simulink model "gm_soc_dvbs2_fpga"  (R2025b)
settings: Solver=VariableStepAuto  StartTime=0.0  StopTime=10.0  RelTol=1e-3
InitFcn:
  | soc_dvbs2_init;
undefined symbols (not defined in the file or in its folder): Add, coefficientsLog, coefficientsSqrt1, coefficientsSqrt2, dataBits, Deinterleaver, designMultirateFIR, noisePow, Shift, Short, soc_dvbs2_designFIRFilter, soc_dvbs2_txPacketBits, syncWord, txDataOut, txFiltCoeff, XData
libraries: simulink x304, hdlsllib x265, dspsigops x15, dsphdlfiltering2 x8, hdlmdlgenlib x6, dsphdlsigops2 x5, commseqgen3 x5, dsphdlmathfun2 x3, hwlogicconnlib x2, whdledac x2, commhdlcrc x2, whdlutilities x1
(part 24 of 36)

== system gm_soc_dvbs2_fpga/DVBS2/DVBS2 TxRx/Channel/AWGN Generator/Unit Variance Gaussian Noise/SinCos/Sine HDL Optimized1/Look-Up Table ==
  In1 : Inport
  Look-Up Table : Lookup_n-D  NumberOfTableDimensions=1  LookupTableObject=''  BreakpointsSpecification=Even spacing  BreakpointsForDimension1=XData  BreakpointsForDimension1FirstPoint="fi(0,0,12,0,\"hex\",\"000\")"  BreakpointsForDimension1Spacing="fi(0,0,12,0,\"hex\",\"001\")"  IndexSearchMethod=Evenly spaced points  Table="fi(\"numerictype\",numerictype(0,15,15),\"Value\",\"[0 0.00152587890625 0.003082275390625 0.004608154296875 0.006134033203125 0.007659912109375 0.00921630859375 0.0107421875 0.01226806640625 0.0137939453125 0.015350341796875 0.016876220703125 0.018402099609375 0.019927978515625 0.021484375 0.02301025390625 0.0245361328125 0.02606201171875 0.027618408203125 0.029144287109375 0.030670166015625 0.032196044921875 0.03375244140625 0.0352783203125 0.03680419921875 0.038330078125 0.039886474609375 0.041412353515625 0.042938232421875 0.044464111328125 0.045989990234375 0.04754638671875 0.049072265625 0.05059814453125 0.0521240234375 0.05364990234375 0.055206298828125 0.056732177734375 0.058258056640625 0.059783935546875 0.061309814453125 0.0628662109375 0.06439208984375 0.06591796875 0.06744384765625 0.0689697265625 0.07049560546875 0.072021484375 0.073577880859375 0.075103759765625 0.076629638671875 0.078155517578125 0.079681396484375 0.081207275390625 0.082733154296875 0.084259033203125 0.085784912109375 0.087310791015625 0.0888671875 0.09039306640625 0.0919189453125 0.09344482421875 0.094970703125 0.09649658203125 0.0980224609375 0.09954833984375 0.10107421875 0.10260009765625 0.1041259765625 0.10565185546875 0.107177734375 0.10870361328125 0.1102294921875 0.11175537109375 0.11328125 0.11480712890625 0.1163330078125 0.117828369140625 0.119354248046875 0.120880126953125 0.122406005859375 0.123931884765625 0.125457763671875 0.126983642578125 0.128509521484375 0.1300048828125 0.13153076171875 0.133056640625 0.13458251953125 0.1361083984375 0.13763427734375 0.139129638671875 0.140655517578125 0.142181396484375 0.143707275390625 0.14520263671875 0.146728515625 0.14825439453125 0.149749755859375 0.151275634765625 0.152801513671875 0.154327392578125 0.15582275390625 0.1573486328125 0.158843994140625 0.160369873046875 0.161895751953125 0.16339111328125 0.1649169921875 0.166412353515625 0.167938232421875 0.169464111328125 0.17095947265625 0.1724853515625 0.173980712890625 0.175506591796875 0.177001953125 0.17852783203125 0.180023193359375 0.1815185546875 0.18304443359375 0.184539794921875 0.186065673828125 0.18756103515625 0.189056396484375 0.190582275390625 0.19207763671875 0.193572998046875 0.195098876953125 0.19659423828125 0.198089599609375 0.199615478515625 0.20111083984375 0.202606201171875 0.2041015625 0.205596923828125 0.207122802734375 0.2086181640625 0.210113525390625 0.21160888671875 0.213104248046875 0.214599609375 0.216094970703125 0.21759033203125 0.2191162109375 0.220611572265625 0.22210693359375 0.223602294921875 0.22509765625 0.226593017578125 0.228057861328125 0.22955322265625 0.231048583984375 0.2325439453125 0.234039306640625 0.23553466796875 0.237030029296875 0.238525390625 0.239990234375 0.241485595703125 0.24298095703125 0.244476318359375 0.245941162109375 0.2474365234375 0.248931884765625 0.25042724609375 0.25189208984375 0.253387451171875 0.254852294921875 0.25634765625 0.257843017578125 0.259307861328125 0.26080322265625 0.26226806640625 0.263763427734375 0.265228271484375 0.2667236328125 0.2681884765625 0.2696533203125 0.271148681640625 0.272613525390625 0.27410888671875 0.27557373046875 0.27703857421875 0.278533935546875 0.279998779296875 0.281463623046875 0.282928466796875 0.284393310546875 0.285888671875 0.287353515625 0.288818359375 0.290283203125 0.291748046875 0.293212890625 0.294677734375 0.296142578125 0.297607421875 0.299072265625 0.300537109375 0.302001953125 0.303466796875 0.304931640625 0.306396484375 0.307861328125 0.309295654296875 0.310760498046875 0.312225341796875 0.313690185546875 0.31512451171875 0.31658935546875 0.31805419921875 0.319488525390625 0.320953369140625 0.322418212890625 0.3238525390625 0.3253173828125 0.326751708984375 0.328216552734375 0.32965087890625 0.33111572265625 0.332550048828125 0.334014892578125 0.33544921875 0.336883544921875 0.338348388671875 0.33978271484375 0.341217041015625 0.3426513671875 0.3441162109375 0.345550537109375 0.34698486328125 0.348419189453125 0.349853515625 0.351287841796875 0.35272216796875 ...(+13376 chars)]\")"  TableDataTypeStr=fixdt(0,15,15)  InterpMethod=Flat  ExtrapMethod=Clip  OutDataTypeStr=fixdt(1,16,15)
  Look-Up Table_pd1 : Delay  DelayLength=1
  Out1 : Outport
  wires:
  In1/1 -> Look-Up Table/1
  Look-Up Table_pd1/1 -> Out1/1
  Look-Up Table/1 -> Look-Up Table_pd1/1

== system gm_soc_dvbs2_fpga/DVBS2/DVBS2 TxRx/Channel/AWGN Generator/Unit Variance Gaussian Noise/SinCos/Sine HDL Optimized2/Look-Up Table ==
  In1 : Inport
  Look-Up Table : Lookup_n-D  NumberOfTableDimensions=1  LookupTableObject=''  BreakpointsSpecification=Even spacing  BreakpointsForDimension1=XData  BreakpointsForDimension1FirstPoint="fi(0,0,12,0,\"hex\",\"000\")"  BreakpointsForDimension1Spacing="fi(0,0,12,0,\"hex\",\"001\")"  IndexSearchMethod=Evenly spaced points  Table="fi(\"numerictype\",numerictype(0,15,15),\"Value\",\"[0 0.00152587890625 0.003082275390625 0.004608154296875 0.006134033203125 0.007659912109375 0.00921630859375 0.0107421875 0.01226806640625 0.0137939453125 0.015350341796875 0.016876220703125 0.018402099609375 0.019927978515625 0.021484375 0.02301025390625 0.0245361328125 0.02606201171875 0.027618408203125 0.029144287109375 0.030670166015625 0.032196044921875 0.03375244140625 0.0352783203125 0.03680419921875 0.038330078125 0.039886474609375 0.041412353515625 0.042938232421875 0.044464111328125 0.045989990234375 0.04754638671875 0.049072265625 0.05059814453125 0.0521240234375 0.05364990234375 0.055206298828125 0.056732177734375 0.058258056640625 0.059783935546875 0.061309814453125 0.0628662109375 0.06439208984375 0.06591796875 0.06744384765625 0.0689697265625 0.07049560546875 0.072021484375 0.073577880859375 0.075103759765625 0.076629638671875 0.078155517578125 0.079681396484375 0.081207275390625 0.082733154296875 0.084259033203125 0.085784912109375 0.087310791015625 0.0888671875 0.09039306640625 0.0919189453125 0.09344482421875 0.094970703125 0.09649658203125 0.0980224609375 0.09954833984375 0.10107421875 0.10260009765625 0.1041259765625 0.10565185546875 0.107177734375 0.10870361328125 0.1102294921875 0.11175537109375 0.11328125 0.11480712890625 0.1163330078125 0.117828369140625 0.119354248046875 0.120880126953125 0.122406005859375 0.123931884765625 0.125457763671875 0.126983642578125 0.128509521484375 0.1300048828125 0.13153076171875 0.133056640625 0.13458251953125 0.1361083984375 0.13763427734375 0.139129638671875 0.140655517578125 0.142181396484375 0.143707275390625 0.14520263671875 0.146728515625 0.14825439453125 0.149749755859375 0.151275634765625 0.152801513671875 0.154327392578125 0.15582275390625 0.1573486328125 0.158843994140625 0.160369873046875 0.161895751953125 0.16339111328125 0.1649169921875 0.166412353515625 0.167938232421875 0.169464111328125 0.17095947265625 0.1724853515625 0.173980712890625 0.175506591796875 0.177001953125 0.17852783203125 0.180023193359375 0.1815185546875 0.18304443359375 0.184539794921875 0.186065673828125 0.18756103515625 0.189056396484375 0.190582275390625 0.19207763671875 0.193572998046875 0.195098876953125 0.19659423828125 0.198089599609375 0.199615478515625 0.20111083984375 0.202606201171875 0.2041015625 0.205596923828125 0.207122802734375 0.2086181640625 0.210113525390625 0.21160888671875 0.213104248046875 0.214599609375 0.216094970703125 0.21759033203125 0.2191162109375 0.220611572265625 0.22210693359375 0.223602294921875 0.22509765625 0.226593017578125 0.228057861328125 0.22955322265625 0.231048583984375 0.2325439453125 0.234039306640625 0.23553466796875 0.237030029296875 0.238525390625 0.239990234375 0.241485595703125 0.24298095703125 0.244476318359375 0.245941162109375 0.2474365234375 0.248931884765625 0.25042724609375 0.25189208984375 0.253387451171875 0.254852294921875 0.25634765625 0.257843017578125 0.259307861328125 0.26080322265625 0.26226806640625 0.263763427734375 0.265228271484375 0.2667236328125 0.2681884765625 0.2696533203125 0.271148681640625 0.272613525390625 0.27410888671875 0.27557373046875 0.27703857421875 0.278533935546875 0.279998779296875 0.281463623046875 0.282928466796875 0.284393310546875 0.285888671875 0.287353515625 0.288818359375 0.290283203125 0.291748046875 0.293212890625 0.294677734375 0.296142578125 0.297607421875 0.299072265625 0.300537109375 0.302001953125 0.303466796875 0.304931640625 0.306396484375 0.307861328125 0.309295654296875 0.310760498046875 0.312225341796875 0.313690185546875 0.31512451171875 0.31658935546875 0.31805419921875 0.319488525390625 0.320953369140625 0.322418212890625 0.3238525390625 0.3253173828125 0.326751708984375 0.328216552734375 0.32965087890625 0.33111572265625 0.332550048828125 0.334014892578125 0.33544921875 0.336883544921875 0.338348388671875 0.33978271484375 0.341217041015625 0.3426513671875 0.3441162109375 0.345550537109375 0.34698486328125 0.348419189453125 0.349853515625 0.351287841796875 0.35272216796875 ...(+13376 chars)]\")"  TableDataTypeStr=fixdt(0,15,15)  InterpMethod=Flat  ExtrapMethod=Clip  OutDataTypeStr=fixdt(1,16,15)
  Look-Up Table_pd1 : Delay  DelayLength=1
  Out1 : Outport
  wires:
  In1/1 -> Look-Up Table/1
  Look-Up Table_pd1/1 -> Out1/1
  Look-Up Table/1 -> Look-Up Table_pd1/1

== system gm_soc_dvbs2_fpga/DVBS2/DVBS2 TxRx/Channel/AWGN Generator/Unit Variance Gaussian Noise/SqrtImplementation/SqrtEval/FunctionEvaluation ==
  x_f : Inport  OutDataTypeStr=fixdt(0, 31, 24)  PortDimensions=1  SampleTime=6.25e-08
  passIn : Inport  Port=2  OutDataTypeStr=fixdt(1, 9, 0)  PortDimensions=1  SampleTime=6.25e-08
  exp_fIn : Inport  Port=3  OutDataTypeStr=int8  PortDimensions=1  SampleTime=6.25e-08
  1-D Lookup Table : Subsystem
  1-D Lookup Table1 : Subsystem
  1-D Lookup Table2 : Subsystem
  1-D Lookup Table3 : Subsystem
  Add : Sum  OutDataTypeStr=fixdt(0, 17, 13)  AccumDataTypeStr=fixdt(1, 44, 36)  SampleTime=6.25e-08
  Add1 : Sum  OutDataTypeStr=fixdt(0, 17, 13)  AccumDataTypeStr=fixdt(0, 17, 13)  SampleTime=6.25e-08
  Constant : Constant  OutDataTypeStr=uint8  SampleTime=6.25e-08
  Constant1 : Constant  Value=2  OutDataTypeStr=uint8  SampleTime=6.25e-08
  Constant2 : Constant  Value=64  OutDataTypeStr=uint8  SampleTime=6.25e-08
  Data Type Conversion : DataTypeConversion  OutDataTypeStr=uint8  SampleTime=6.25e-08  SaturateOnIntegerOverflow=off  RndMeth=Floor
  Data Type Conversion1 : DataTypeConversion  OutDataTypeStr=uint8  SampleTime=6.25e-08  SaturateOnIntegerOverflow=off  RndMeth=Floor
  Delay{,1..7,9..10,13..14} (12 alike) : Delay  DelayLength=double(1)  InitialCondition=0  SampleTime=6.25e-08
  Delay{8,11..12,15..25} (14 alike) : Delay  DelayLength=double(2)  InitialCondition=0  SampleTime=6.25e-08
  Product : Product  Inputs=**  OutDataTypeStr=fixdt(1, 44, 36)  SampleTime=6.25e-08
  Product1 : Product  Inputs=**  OutDataTypeStr=fixdt(1, 44, 36)  SampleTime=6.25e-08
  Shift Arithmetic1 : ArithShift  BitShiftNumber=double(0)  BinPtShiftNumber=double(6)
  Shift Arithmetic2 : ArithShift  BitShiftNumber=double(0)  BinPtShiftNumber=double(5)
  Subtract : Sum  Inputs=+-  OutDataTypeStr=fixdt(1, 33, 24)  AccumDataTypeStr=fixdt(1, 33, 24)  SampleTime=6.25e-08
  Subtract1 : Sum  Inputs=+-  OutDataTypeStr=fixdt(0, 31, 24)  AccumDataTypeStr=fixdt(0, 31, 24)  SampleTime=6.25e-08
  Switch : Switch  Criteria=u2 ~= 0  Threshold="fi(0,1,9,0,\"hex\",\"000\")"  OutDataTypeStr=fixdt(0, 17, 13)  SampleTime=6.25e-08  SaturateOnIntegerOverflow=off  InputSameDT=off
  Switch1 : Switch  Criteria=u2 > Threshold  Threshold="fi(0,0,8,0,\"hex\",\"3f\")"  OutDataTypeStr=uint8  SampleTime=6.25e-08  SaturateOnIntegerOverflow=off  InputSameDT=off
  Switch2 : Switch  Criteria=u2 > Threshold  Threshold="fi(0,0,8,0,\"hex\",\"3f\")"  OutDataTypeStr=int8  SampleTime=6.25e-08  SaturateOnIntegerOverflow=off  InputSameDT=off
  y_f : Outport  SampleTime=6.25e-08
  passOut : Outport  Port=2  SampleTime=6.25e-08
  exp_fOut : Outport  Port=3  SampleTime=6.25e-08
  wires:
  Constant1/1 -> Subtract1/2
  Constant/1 -> Subtract/2
  Constant2/1 -> Switch2/1, Switch1/1
  exp_fIn/1 -> Delay7/1
  Shift Arithmetic2/1 -> Data Type Conversion1/1
  Subtract1/1 -> Shift Arithmetic2/1
  Subtract/1 -> Shift Arithmetic1/1
  x_f/1 -> Delay4/1, Subtract1/1, Delay/1, Subtract/1
  Delay7/1 -> Delay15/1
  Delay16/1 -> Add/1
  Delay/1 -> Delay8/1
  Delay15/1 -> Delay21/1
  Switch/1 -> y_f/1
  Shift Arithmetic1/1 -> Data Type Conversion/1
  Delay2/1 -> 1-D Lookup Table1/1(In1)
  Delay4/1 -> Delay12/1
  Delay21/1 -> Delay25/1
  Delay8/1 -> Product/1
  passIn/1 -> Delay3/1
  Data Type Conversion/1 -> Switch1/3, Switch1/2
  Switch1/1 -> Delay2/1, Delay1/1
  Data Type Conversion1/1 -> Switch2/3, Switch2/2
  Delay18/1 -> Delay23/1
  Delay25/1 -> exp_fOut/1
  Delay12/1 -> Product1/1
  Switch2/1 -> Delay6/1, Delay5/1
  Delay17/1 -> Add/2
  Delay1/1 -> 1-D Lookup Table/1(In1)
  Product/1 -> Delay16/1
  Delay5/1 -> 1-D Lookup Table2/1(In1)
  1-D Lookup Table/1(Out1) -> Delay9/1
  Delay6/1 -> 1-D Lookup Table3/1(In1)
  1-D Lookup Table2/1(Out1) -> Delay13/1
  1-D Lookup Table1/1(Out1) -> Delay10/1
  1-D Lookup Table3/1(Out1) -> Delay14/1
  Product1/1 -> Delay19/1
  Delay9/1 -> Product/2
  Delay10/1 -> Delay17/1
  Delay13/1 -> Product1/2
  Delay14/1 -> Delay20/1
  Delay19/1 -> Add1/1
  Delay3/1 -> Delay11/1
  Delay20/1 -> Add1/2
  Delay11/1 -> Delay18/1
  Add/1 -> Delay22/1
  Add1/1 -> Delay24/1
  Delay22/1 -> Switch/1
  Delay24/1 -> Switch/3
  Delay23/1 -> passOut/1, Switch/2

== system gm_soc_dvbs2_fpga/DVBS2/DVBS2 TxRx/Channel/AWGN Generator/Unit Variance Gaussian Noise/SqrtImplementation/SqrtEval/RangeReconstruction ==
  y_f : Inport  OutDataTypeStr=fixdt(0, 17, 13)  PortDimensions=1  SampleTime=6.25e-08
  pass : Inport  Port=2  OutDataTypeStr=fixdt(1, 9, 0)  PortDimensions=1  SampleTime=6.25e-08
  exp_f : Inport  Port=3  OutDataTypeStr=int8  PortDimensions=1  SampleTime=6.25e-08
  Add : Sum  OutDataTypeStr=int8  AccumDataTypeStr=int8
  Constant : Constant  OutDataTypeStr=int8  SampleTime=-1
  Delay{1..3,8} (4 alike) : Delay
  Delay{4..7,9..12} (8 alike) : Delay  DelayLength=1
  Gain : Gain  Gain=-1  OutDataTypeStr=int8
  Shift Arithmetic : ArithShift  BitShiftNumber=1
  Shift Arithmetic1 : ArithShift  BitShiftNumberSource=Input port  BitShiftNumber=8
      settings: InputPortMap=u0,p1
  Switch : Switch  Criteria=u2 ~= 0  OutDataTypeStr=int8  SaturateOnIntegerOverflow=off  InputSameDT=off
  f : Outport  SampleTime=6.25e-08
  wires:
  y_f/1 -> Delay9/1
  Delay12/1 -> Delay6/1
  Delay11/1 -> Delay7/1
  Delay2/1 -> Gain/1
  pass/1 -> Delay11/1
  Delay10/1 -> Add/2
  Constant/1 -> Add/1
  exp_f/1 -> Delay12/1, Delay10/1
  Delay4/1 -> Switch/1
  Delay6/1 -> Switch/3
  Add/1 -> Delay4/1
  Delay7/1 -> Switch/2
  Switch/1 -> Shift Arithmetic/1
  Delay9/1 -> Delay5/1
  Shift Arithmetic/1 -> Delay2/1
  Delay5/1 -> Delay3/1
  Delay3/1 -> Delay1/1
  Gain/1 -> Delay8/1
  Delay1/1 -> Shift Arithmetic1/1
  Shift Arithmetic1/1 -> f/1
  Delay8/1 -> Shift Arithmetic1/2

== system gm_soc_dvbs2_fpga/DVBS2/DVBS2 TxRx/Channel/AWGN Generator/Unit Variance Gaussian Noise/SqrtImplementation/SqrtEval/RangeReduction ==
  note: Range of x_f=[1,4)
  u : Inport  OutDataTypeStr=fixdt(0, 31, 24)  PortDimensions=1  SampleTime=6.25e-08
  Add : Sum  Inputs=+-  OutDataTypeStr=int8
  Constant : Constant  Value=5  OutDataTypeStr=uint8  SampleTime=-1
  Data Type Conversion : DataTypeConversion  OutDataTypeStr=fixdt(0,38,31)  SaturateOnIntegerOverflow=off  RndMeth=Floor
  Delay{1..20} (20 alike) : Delay  DelayLength=1
  Shift Arithmetic : ArithShift  BitShiftNumberSource=Input port  BitShiftNumber=8
      settings: InputPortMap=u0,p1
  Shift Arithmetic1 : ArithShift  BitShiftNumber=1  BitShiftDirection=Right
  Shift Arithmetic2 : ArithShift  BitShiftNumber=6  BitShiftDirection=Right
  Shift Arithmetic3 : ArithShift  BitShiftNumber=1  BitShiftDirection=Right
  Shift Arithmetic4 : ArithShift  BitShiftNumber=1  BitShiftDirection=Left
  Subtract : Sum  Inputs=+-  OutDataTypeStr=fixdt(1, 9, 0)
  Switch : Switch  Criteria=u2 ~= 0  OutDataTypeStr=fixdt(0, 31, 24)  SaturateOnIntegerOverflow=off  InputSameDT=off
  leadingZeroDetector : MATLAB Function  TreatAsAtomicUnit=on
  x_f : Outport  SampleTime=6.25e-08
  pass : Outport  Port=2  SampleTime=6.25e-08
  exp_f : Outport  Port=3  SampleTime=6.25e-08  VectorParamsAs1DForOutWhenUnconnected=off
  wires:
  u/1 -> Data Type Conversion/1, Delay3/1
  Delay20/1 -> leadingZeroDetector/1(x)
  Delay8/1 -> Subtract/1
  Delay19/1 -> Delay13/1
  Delay9/1 -> Subtract/2
  Delay2/1 -> Delay19/1
  Delay3/1 -> Delay2/1
  Shift Arithmetic2/1 -> Delay20/1
  Shift Arithmetic4/1 -> Delay9/1
  Data Type Conversion/1 -> Shift Arithmetic2/1
  leadingZeroDetector/1(exp_f) -> Delay4/1
  Delay16/1 -> Shift Arithmetic4/1
  Constant/1 -> Add/1
  Delay4/1 -> Add/2
  Delay13/1 -> Shift Arithmetic/1
  Shift Arithmetic3/1 -> Delay16/1
  Add/1 -> Delay18/1
  Delay10/1 -> Delay7/1
  Delay18/1 -> Shift Arithmetic3/1, Delay15/1, Delay14/1, Delay17/1
  Delay14/1 -> Shift Arithmetic/2
  Delay1/1 -> Switch/1
  Delay17/1 -> Delay10/1
  Delay15/1 -> Delay8/1
  Subtract/1 -> Delay6/1
  Shift Arithmetic/1 -> Delay11/1, Delay12/1
  Delay7/1 -> exp_f/1
  Delay12/1 -> Shift Arithmetic1/1
  Shift Arithmetic1/1 -> Delay1/1
  Delay11/1 -> Delay5/1
  Delay5/1 -> Switch/3
  Delay6/1 -> Switch/2, pass/1
  Switch/1 -> x_f/1

== system gm_soc_dvbs2_fpga/DVBS2/DVBS2 TxRx/Channel/AWGN Generator/Unit Variance Gaussian Noise/logImplementation/log/FunctionEvaluation ==
  x_e : Inport  OutDataTypeStr=fixdt(0, 49, 48)  PortDimensions=1  SampleTime=6.25e-08
  exp_eIn : Inport  Port=2  OutDataTypeStr=uint8  PortDimensions=1  SampleTime=6.25e-08
  1-D Lookup Table : Lookup_n-D  NumberOfTableDimensions=1  LookupTableObject=''  BreakpointsForDimension1=0:255  BreakpointsForDimension1FirstPoint=10  BreakpointsForDimension2FirstPoint=10  BreakpointsForDimension1Spacing=12  BreakpointsForDimension2Spacing=12  IndexSearchMethod=Evenly spaced points  Table=coefficientsLog(:,1)  InterpMethod=Flat  InternalRulePriority=Speed  OutDataTypeStr=fixdt(1,16,15)  RndMeth=Simplest
  1-D Lookup Table1 : Lookup_n-D  NumberOfTableDimensions=1  LookupTableObject=''  BreakpointsForDimension1=0:255  BreakpointsForDimension1FirstPoint=10  BreakpointsForDimension2FirstPoint=10  BreakpointsForDimension1Spacing=12  BreakpointsForDimension2Spacing=12  IndexSearchMethod=Evenly spaced points  Table=coefficientsLog(:,2)  InterpMethod=Flat  InternalRulePriority=Speed  OutDataTypeStr=fixdt(1,16,14)  RndMeth=Simplest
  1-D Lookup Table2 : Lookup_n-D  NumberOfTableDimensions=1  LookupTableObject=''  BreakpointsForDimension1=0:255  BreakpointsForDimension1FirstPoint=10  BreakpointsForDimension2FirstPoint=10  BreakpointsForDimension1Spacing=12  BreakpointsForDimension2Spacing=12  IndexSearchMethod=Evenly spaced points  Table=coefficientsLog(:,3)  InterpMethod=Flat  InternalRulePriority=Speed  OutDataTypeStr=fixdt(1,32,30)  RndMeth=Simplest
  Add : Sum  OutDataTypeStr=fixdt(1, 16, 14)  AccumDataTypeStr=fixdt(1, 18, 15)  SampleTime=6.25e-08
  Add1 : Sum  OutDataTypeStr=fixdt(1, 31, 27)  AccumDataTypeStr=fixdt(1, 35, 30)  SampleTime=6.25e-08
  Data Type Conversion : DataTypeConversion  OutDataTypeStr=uint8  SampleTime=6.25e-08  SaturateOnIntegerOverflow=off  RndMeth=Floor
  Data Type Conversion1 : DataTypeConversion  OutDataTypeStr=fixdt(0, 16, 15)  SampleTime=6.25e-08  SaturateOnIntegerOverflow=off  RndMeth=Floor
  Delay1 : Delay  DelayLength=double(1)  InitialCondition=0  SampleTime=6.25e-08
  Delay{3..30} (28 alike) : Delay  DelayLength=double(2)  InitialCondition=0  SampleTime=6.25e-08
  Delay2 : Delay  DelayLength=double(1)  InitialCondition=0  SampleTime=6.25e-08
  Product : Product  Inputs=**  OutDataTypeStr=fixdt(1, 32, 30)  SampleTime=6.25e-08
  Product1 : Product  Inputs=**  OutDataTypeStr=fixdt(1, 32, 29)  SampleTime=6.25e-08
  Product1_out_dtc : DataTypeConversion  OutDataTypeStr=fixdt(1, 31, 27)  SampleTime=6.25e-08  SaturateOnIntegerOverflow=off  RndMeth=Floor
  Product_out_dtc : DataTypeConversion  OutDataTypeStr=fixdt(1, 16, 15)  SampleTime=6.25e-08  SaturateOnIntegerOverflow=off  RndMeth=Floor
  Shift Arithmetic1 : ArithShift  BitShiftNumber=double(0)  BinPtShiftNumber=double(8)
  y_e : Outport  SampleTime=6.25e-08
  exp_eOut : Outport  Port=2  SampleTime=6.25e-08
  wires:
  Delay10/1 -> Add/1
  x_e/1 -> Shift Arithmetic1/1, Data Type Conversion1/1
  Delay11/1 -> Delay6/1
  exp_eIn/1 -> Delay30/1
  Delay9/1 -> Delay5/1
  Delay29/1 -> Delay20/1
  Delay30/1 -> Delay29/1
  Data Type Conversion/1 -> Delay28/1, Delay27/1, Delay24/1
  Data Type Conversion1/1 -> Delay23/1
  Shift Arithmetic1/1 -> Data Type Conversion/1
  Delay23/1 -> Delay21/1
  Delay28/1 -> 1-D Lookup Table2/1
  Delay20/1 -> Delay14/1
  Delay24/1 -> 1-D Lookup Table/1
  Delay2/1 -> exp_eOut/1
  Delay27/1 -> 1-D Lookup Table1/1
  Delay14/1 -> Delay9/1
  Add/1 -> Delay7/1
  1-D Lookup Table/1 -> Delay22/1  "c2"
  1-D Lookup Table1/1 -> Delay25/1  "c1"
  1-D Lookup Table2/1 -> Delay26/1  "c0"
  Delay21/1 -> Delay15/1, Delay17/1
  Delay22/1 -> Delay16/1
  Delay26/1 -> Delay19/1
  Product/1 -> Product_out_dtc/1
  Delay5/1 -> Delay2/1
  Delay17/1 -> Delay11/1
  Delay15/1 -> Product/1
  Delay16/1 -> Product/2
  Delay25/1 -> Delay18/1
  Delay18/1 -> Delay12/1
  Delay19/1 -> Delay13/1
  Product_out_dtc/1 -> Delay10/1
  Delay12/1 -> Add/2
  Delay13/1 -> Delay8/1
  Delay8/1 -> Delay4/1
  Delay6/1 -> Product1/1
  Delay7/1 -> Product1/2
  Delay4/1 -> Add1/2
  Product1/1 -> Product1_out_dtc/1
  Add1/1 -> Delay1/1
  Product1_out_dtc/1 -> Delay3/1
  Delay3/1 -> Add1/1
  Delay1/1 -> y_e/1
